simulink model "test"  (R2021a)
settings: Solver=VariableStepAuto  StartTime=0.0  StopTime=10.0  RelTol=1e-3
values from neighbouring files (symbols this model uses):
  F_A = dcgain(H_c_A)^-1    [SupportFile.m]
  F_E = dcgain(H_c_E)^-1    [SupportFile.m]
  F_R = dcgain(H_c_R)^-1    [SupportFile.m]
  F_T = dcgain(H_c_T)^-1    [SupportFile.m]
  K_A = place(A_A, B_A, [-5 -2 -1])    [SupportFile.m]
  K_E = place(A_E, B_E, [-5 -2 -1])    [SupportFile.m]
  K_R = place(A_R, B_R, [-5 -2])    [SupportFile.m]
  K_T = place(A_T, B_T, [-5 -2])    [SupportFile.m]
undefined symbols (not defined in the file or in its folder): g, m
settings Model: Creator=hukai  LastModifiedBy=hukai

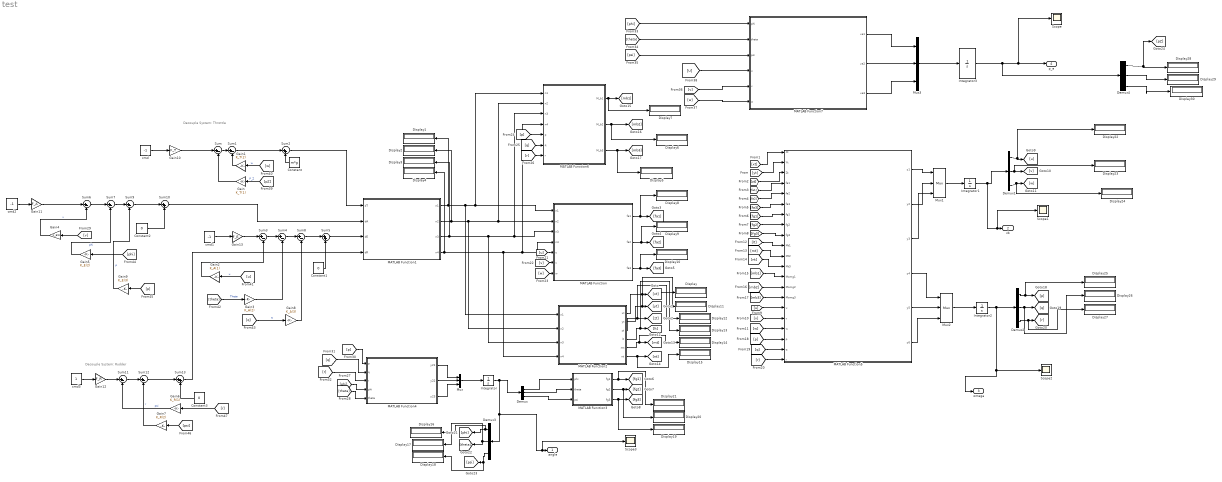
== system test ==
  note: Decouple System: Throttle
  note: Decouple System: Rudder
  Constant : Constant  Value=m*g
  Constant1 : Constant  Value=0
  Constant2 : Constant  Value=0
  Constant3 : Constant  Value=0
  Demux{,1..4} (5 alike) : Demux  Outputs=3
  Display{,1..30} (31 alike) : Display
  Gain : Gain  Gain=K_T(1)
  Gain1 : Gain  Gain=K_T(2)
  Gain10 : Gain  Gain=F_T
  Gain11 : Gain  Gain=F_A
  Gain12 : Gain  Gain=F_R
  Gain13 : Gain  Gain=F_E
  Gain2 : Gain  Gain=K_A(1)
  Gain3 : Gain  Gain=K_A(2)
  Gain4 : Gain  Gain=K_E(1)
  Gain5 : Gain  Gain=K_E(2)
  Gain6 : Gain  Gain=K_R(1)
  Gain7 : Gain  Gain=K_R(2)
  Gain8 : Gain  Gain=K_A(3)
  Gain9 : Gain  Gain=K_E(3)
  Integrator{,1..3} (4 alike) : Integrator  InitialCondition=[0;0;0]
  MATLAB Function : MATLAB Function  Tag=Aerodynamic Forces and Moments  TreatAsAtomicUnit=on
      settings: AttributesFormatString=%<Tag>
  MATLAB Function1 : MATLAB Function  Tag=Mixer  TreatAsAtomicUnit=on
      settings: AttributesFormatString=%<Tag>
  MATLAB Function2 : MATLAB Function  Tag=Propulsive Motor Forces and Moments  TreatAsAtomicUnit=on
      settings: AttributesFormatString=%<Tag>
  MATLAB Function3 : MATLAB Function  Tag=Model Gravity  TreatAsAtomicUnit=on
      settings: AttributesFormatString=%<Tag>
  MATLAB Function4 : MATLAB Function  Tag=Rotational Kinmeatics  TreatAsAtomicUnit=on
      settings: AttributesFormatString=%<Tag>
  MATLAB Function5 : MATLAB Function  TreatAsAtomicUnit=on
  MATLAB Function6 : MATLAB Function  Tag=Gyroscopic Forces and Moments  TreatAsAtomicUnit=on
      settings: AttributesFormatString=%<Tag>
  MATLAB Function7 : MATLAB Function  TreatAsAtomicUnit=on
  Mux{,1..3} (4 alike) : Mux  Inputs=3
  Scope{,1..3} (4 alike) : Scope
  Sum{,1,3..4,6..9,11..12} (10 alike) : Sum  Inputs=|+-
  Sum{2,5,10,13} (4 alike) : Sum  Inputs=|++
  cmd : Constant  Value=-1
  cmd1 : Constant  Value=-1
  cmd2 : Constant  Value=-1
  cmd3 : Constant
  angle : Outport
  vb : Outport  Port=2
  omega : Outport  Port=3
  p_e : Outport  Port=4
  wires:
  MATLAB Function7/1(ve1) -> Mux3/1
  [mb3] -> MATLAB Function5/15(Momg3)
  [w] -> MATLAB Function7/6(w)
  Demux2/2 -> Display26/1, [q]
  [mb1] -> MATLAB Function5/13(Momg1)
  MATLAB Function3/3(fg3) -> Display19/1, [fg3]
  MATLAB Function6/1(M_b1) -> Display7/1, [mb1]
  MATLAB Function4/3(y23) -> Mux/3
  [mt] -> MATLAB Function5/11(Mt2)
  MATLAB Function/3(fa3) -> Display10/1, [fa3]
  Mux/1 -> Integrator/1
  Demux/3 -> MATLAB Function3/3(psi)
  MATLAB Function4/1(y21) -> Mux/1
  MATLAB Function3/1(fg1) -> Display21/1, [fg1]
  [fa2] -> MATLAB Function5/5(fa2)
  [lt] -> MATLAB Function5/10(Mt1)
  MATLAB Function2/1(xt) -> Display/1, [xt]
  Demux1/1 -> Display22/1, [u]
  MATLAB Function2/5(mt) -> Display14/1, [mt]
  [fg1] -> MATLAB Function5/7(fg1)
  MATLAB Function2/6(nt) -> Display15/1, [nt]
  MATLAB Function5/1(y1) -> Mux1/1
  [w] -> MATLAB Function5/18(w)
  Demux1/3 -> Display24/1, [w]
  [fg3] -> MATLAB Function5/9(fg3)
  [u] -> MATLAB Function5/16(u)
  Integrator1/1 -> Scope1/1, vb/1, Demux1/1
  MATLAB Function1/4(n4) -> MATLAB Function2/4(n4), MATLAB Function6/4(n4), MATLAB Function/4(n4), Display4/1
  MATLAB Function3/2(fg2) -> Display20/1, [fg2]
  [fg2] -> MATLAB Function5/8(fg2)
  MATLAB Function5/5(y5) -> Mux2/2
  [fa3] -> MATLAB Function5/6(fa3)
  [v] -> MATLAB Function5/17(v)
  Demux1/2 -> Display23/1, [v]
  Mux1/1 -> Integrator1/1
  [xt] -> MATLAB Function5/1(Xt)
  MATLAB Function/2(fa2) -> Display9/1, [fa2]
  MATLAB Function/1(fa1) -> Display8/1, [fa1]
  [zt] -> MATLAB Function5/3(Zt)
  MATLAB Function2/3(zt) -> Display12/1, [zt]
  MATLAB Function5/6(y6) -> Mux2/3
  MATLAB Function1/1(n1) -> Display1/1, MATLAB Function2/1(n1), MATLAB Function6/1(n1), MATLAB Function/1(n1)
  MATLAB Function2/2(yt) -> Display11/1, [yt]
  [yt] -> MATLAB Function5/2(Yt)
  MATLAB Function5/2(y2) -> Mux1/2
  Demux/2 -> MATLAB Function3/2(theta)
  Demux/1 -> MATLAB Function3/1(phi)
  Demux3/3 -> Display18/1, [psi]
  MATLAB Function5/4(y4) -> Mux2/1
  [q] -> MATLAB Function6/6(q)
  [r] -> MATLAB Function6/7(r)
  [w] -> MATLAB Function/7(w)
  MATLAB Function7/2(ve2) -> Mux3/2
  [p] -> MATLAB Function4/1(p)
  Integrator3/1 -> Demux4/1, Scope/1, p_e/1
  MATLAB Function5/3(y3) -> Mux1/3
  Integrator/1 -> Scope3/1, angle/1, Demux3/1, Demux/1
  MATLAB Function4/2(y22) -> Mux/2
  [theta] -> MATLAB Function4/5(theta)
  MATLAB Function1/3(n3) -> Display3/1, MATLAB Function2/3(n3), MATLAB Function6/3(n3), MATLAB Function/3(n3)
  Demux3/1 -> Display16/1, [phi]
  Demux2/1 -> Display25/1, [p]
  [psi] -> MATLAB Function7/3(psi)
  [v] -> MATLAB Function/6(v)
  Mux3/1 -> Integrator3/1
  [phi] -> MATLAB Function7/1(phi)
  [r] -> MATLAB Function4/3(r)
  [theta] -> MATLAB Function7/2(theta)
  [p] -> MATLAB Function5/19(p)
  [u] -> MATLAB Function/5(u)
  [phi] -> MATLAB Function4/4(phi)
  Mux2/1 -> Integrator2/1
  MATLAB Function6/3(M_b3) -> Display5/1, [mb3]
  Demux3/2 -> [theta], Display17/1
  [v] -> MATLAB Function7/5(v)
  [p] -> MATLAB Function6/5(p)
  [u] -> MATLAB Function7/4(u)
  MATLAB Function1/2(n2) -> Display2/1, MATLAB Function2/2(n2), MATLAB Function6/2(n2), MATLAB Function/2(n2)
  MATLAB Function7/3(ve3) -> Mux3/3
  MATLAB Function2/4(lt) -> Display13/1, [lt]
  [nt] -> MATLAB Function5/12(Mt3)
  [mb2] -> MATLAB Function5/14(Momg2)
  [q] -> MATLAB Function5/20(q)
  [q] -> MATLAB Function4/2(q)
  Demux2/3 -> Display27/1, [r]
  MATLAB Function6/2(M_b2) -> Display6/1, [mb2]
  [fa1] -> MATLAB Function5/4(fa1)
  [r] -> MATLAB Function5/21(r)
  Integrator2/1 -> Scope2/1, omega/1, Demux2/1
  Demux4/1 -> [pZ], Display28/1
  Demux4/2 -> Display29/1
  Demux4/3 -> Display30/1
  cmd/1 -> Gain10/1
  Gain10/1 -> Sum/1
  [pZ] -> Gain/1  "P_Z"
  Gain/1 -> Sum/2
  [w] -> Gain1/1  "w"
  Gain1/1 -> Sum1/2
  Sum/1 -> Sum1/1
  Sum1/1 -> Sum2/1
  Constant/1 -> Sum2/2
  Sum2/1 -> MATLAB Function1/1(dT)
  Sum4/1 -> Sum8/1
  Gain2/1 -> Sum3/2
  [q] -> Gain8/1  "q"
  Sum3/1 -> Sum4/1
  [u] -> Gain2/1  "u"
  Gain3/1 -> Sum4/2
  Gain8/1 -> Sum8/2
  [theta] -> Gain3/1  "Theta"
  Sum8/1 -> Sum5/1
  Constant1/1 -> Sum5/2
  Sum9/1 -> Sum10/1
  [p] -> Gain9/1
  Gain4/1 -> Sum6/2  "v"
  Gain9/1 -> Sum9/2  "p"
  Gain5/1 -> Sum7/2  "phi"
  [v] -> Gain4/1
  Sum7/1 -> Sum9/1
  Sum6/1 -> Sum7/1
  [phi] -> Gain5/1
  cmd1/1 -> Gain13/1
  Gain13/1 -> Sum3/1
  Sum5/1 -> MATLAB Function1/3(dE)
  cmd2/1 -> Gain11/1
  Gain11/1 -> Sum6/1
  Constant2/1 -> Sum10/2
  Sum10/1 -> MATLAB Function1/2(dA)
  Gain6/1 -> Sum11/2  "psi"
  Sum11/1 -> Sum12/1
  [psi] -> Gain7/1
  Gain12/1 -> Sum11/1
  Sum12/1 -> Sum13/1
  cmd3/1 -> Gain12/1
  [r] -> Gain6/1
  Gain7/1 -> Sum12/2  "r"
  Constant3/1 -> Sum13/2
  Sum13/1 -> MATLAB Function1/4(dR)

== matlab function test/MATLAB Function6 ==
  data: n1 input; M_b1 output; n2 input; n3 input; n4 input; p input; q input; r input; M_b2 output; M_b3 output
function [M_b1,M_b2,M_b3] = fcn12(n1,n2,n3,n4,p,q,r)
Jp=1.0207e-05;
hb = Jp*2*pi*(n1-n2+n3-n4);
Hb = [0;0;hb];
omega = [p;q;r];
Mb = cross(Hb,omega);
M_b1 = Mb(1);
M_b2 = Mb(2);
M_b3 = Mb(3);

== matlab function test/MATLAB Function7 ==
  data: phi input; theta input; psi input; u input; ve1 output; v input; w input; ve2 output; ve3 output
function [ve1,ve2,ve3] = fcn10(phi,theta,psi,u,v,w)
cpsi = cos(psi);
spsi = sin(psi);
R_psi = [ cpsi spsi 0    ;...
          -spsi cpsi 0  ;...
          0 0 1  ];
cphi = cos(phi);
sphi = sin(phi);
R_phi = [ 1 0 0    ;...
          0 cphi sphi  ;...
          0 -sphi cphi  ];

ctheta = cos(theta);
stheta = sin(theta);
R_theta = [ ctheta 0 -stheta       ;....
            0 1  0 ;....
            stheta 0 ctheta ];
F_b = R_phi *  R_theta * R_psi;
v_b = [u;v;w];
v_e = F_b\v_b;
ve1 = v_e(1);
ve2 = v_e(2);
ve3 = v_e(3);

== matlab function test/MATLAB Function ==
  data: n1 input; n2 input; n3 input; n4 input; u input; fa1 output; v input; w input; fa2 output; fa3 output
function [fa1,fa2,fa3] = fcn11(n1,n2,n3,n4,u,v,w)
v_b = [u;v;w];
a = 1.948E-6;
kc = 0.22;
K_c = [kc 0 0;
    0 kc 0;
    0 0 0];
F_b = -a*(n1^2+n2^2+n3^2+n4^2)*K_c*v_b;
fa1 = F_b(1);
fa2 = F_b(2);
fa3 = F_b(3);

== matlab function test/MATLAB Function1 ==
  data: dT input; n1 output; dA input; dE input; dR input; n2 output; n3 output; n4 output
function [n1,n2,n3,n4] = fcn9(dT,dA,dE,dR)
a = 1.948E-6;
b = 9.277E-8;
c = 9.277E-8;
d=1.017E-7;
input = [dT;dA;dE;dR];
coeff = [a 0 0 0;
    0 b 0 0;
    0 0 c 0;
    0 0 0 d;];
ones_1 = [1 1 1 1;
    1 -1 -1 1;
    1 1 -1 -1;
    -1 1 -1 1;];
coeff1 = coeff*ones_1;
v_final1 = inv(coeff1)*input;
v_final = abs(v_final1);
n1 = sqrt(v_final(1))
n2 = sqrt(v_final(2));
n3 = sqrt(v_final(3));
n4 = sqrt(v_final(4));

== matlab function test/MATLAB Function2 ==
  data: n1 input; xt output; n2 input; n3 input; n4 input; yt output; zt output; lt output; mt output; nt output
function [xt,yt,zt,lt,mt,nt] = fcn8(n1,n2,n3,n4)
a = 1.948E-6;
b = 9.277E-8;
c = 9.277E-8;
d=1.017E-7;
xt = 0;
yt = 0;
zt = -a*(n1^2+n2^2+n3^2+n4^2);
lt = b*(n1^2-n2^2-n3^2+n4^2);
mt = c*(n1^2+n2^2-n3^2-n4^2);
nt = d*(-n1^2+n2^2-n2^3+n4^2);

== matlab function test/MATLAB Function3 ==
  data: phi input; fg1 output; theta input; fg2 output; psi input; fg3 output
function [fg1,fg2,fg3] = fcn2(phi,theta,psi)
g = 9.81;
m = .068;
cpsi = cos(psi);
spsi = sin(psi);
R_psi = [ cpsi spsi 0    ;...
          -spsi cpsi 0  ;...
          0 0 1  ];

cphi = cos(phi);
sphi = sin(phi);
R_phi = [ 1 0 0    ;...
          0 cphi sphi  ;...
          0 -sphi cphi  ];

ctheta = cos(theta);
stheta = sin(theta);
R_theta = [ ctheta 0 -stheta       ;....
            0 1  0 ;....
            stheta 0 ctheta ];
F_g_b = R_phi *  R_theta* R_psi;
fe = [0;0;m*g];
fb = F_g_b*fe;
fg1 = fb(1);
fg2 = fb(2);
fg3 = fb(3);

== matlab function test/MATLAB Function4 ==
  data: y21 output; p input; q input; r input; y22 output; y23 output; phi input; theta input
function [y21,y22,y23] = fcn2(p,q,r,phi,theta)
omega = [p;q;r];
dotangle = [1, (sin(phi)*sin(theta))/cos(theta), (cos(phi)*sin(theta))/cos(theta);...
0,                         cos(phi),                        -sin(phi);...
0,              sin(phi)/cos(theta),              cos(phi)/cos(theta)]*omega;
y21 = dotangle(1);
y22 = dotangle(2);
y23 = dotangle(3);

== matlab function test/MATLAB Function5 ==
  data: Xt input; Yt input; Zt input; fa1 input; fa2 input; fa3 input; fg1 input; fg2 input; fg3 input; Mt1 input; Mt2 input; Mt3 input; Momg1 input; Momg2 input; Momg3 input; u input; y1 output; v input; w input; p input; q input; r input; y2 output; y3 output; y4 output; y5 output; y6 output
function [y1,y2,y3,y4,y5,y6] = func1(Xt,Yt,Zt,fa1,fa2,fa3,fg1,fg2,fg3,Mt1,Mt2,Mt3,Momg1,Momg2,Momg3,u,v,w,p,q,r)
m=0.068;
Jxx = 0.69E-4;
Jyy = 0.77E-4;
Jzz = 1.5E-4;
J = [Jxx 0 0 ;
    0 Jyy 0;
    0 0 Jzz];
F_t = [Xt;Yt;Zt];
F_a = [fa1;fa2;fa3];
F_g = [fg1;fg2;fg3];
M_t = [Mt1;Mt2;Mt3];
M_a = [0;0;0];
M_omg = [Momg1;Momg2;Momg3];
V_b = [u;v;w];
Omega = [p;q;r];
dotV = (1/m).*(F_t+F_a+F_g-cross(Omega,m.*V_b));
dotOmega = (M_t+M_a+M_omg-cross(Omega,J*Omega))\J;
y1 = dotV(1);
y2 = dotV(2);
y3 = dotV(3);
y4 = dotOmega(1);
y5 = dotOmega(2);
y6 = dotOmega(3);
